simulink model "MBDMotorSystemModel"  (R2023a)
settings: Solver=VariableStepAuto  StartTime=0.0  StopTime=1  RelTol=1e-3
undefined symbols (not defined in the file): CntFdqDcpMap, CntLdqDMap, CntTrqReqMap, DiscIntNeverNeededParam, MdlFluxMap, MdlTrqMap, Pos0
libraries: simulink x29, simulink_extras x6
(part 1 of 3)
settings Model: SimulationMode=accelerator  Creator=DevMDG39khtN  LastModifiedBy=DevMDG39khtN

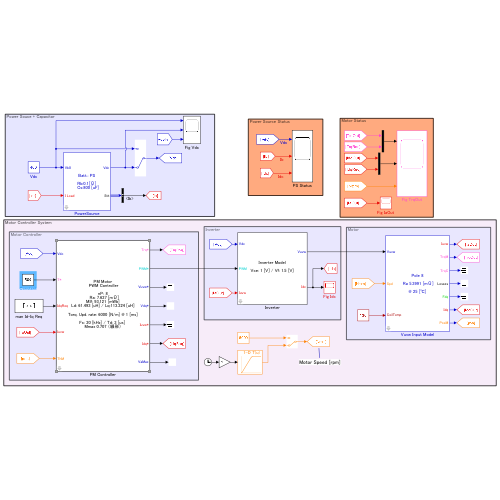
[thumbnail: Simulink's stored preview of the top-level diagram]
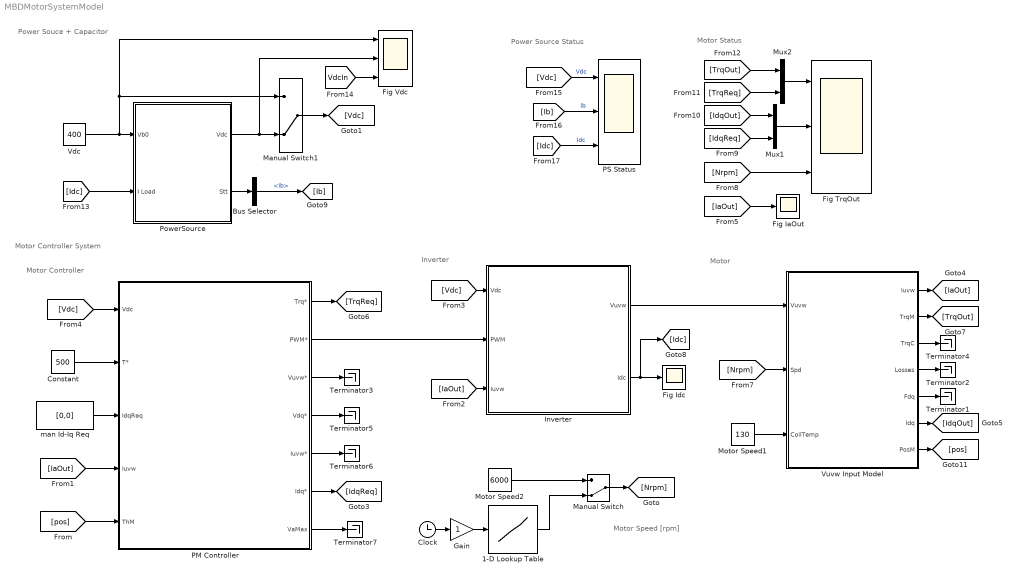
== system MBDMotorSystemModel ==
  note: Motor Speed [rpm]
  note: Power Source Status
  note: Motor Controller System
  note: Motor Controller
  note: Inverter
  note: Motor
  note: Motor Status
  note: Power Souce + Capacitor
  1-D Lookup Table : Lookup_n-D  NumberOfTableDimensions=1  BreakpointsForDimension1=[0 0.01 0.4 0.45 0.8]  Table=[0 0 12000 13000 13000]  InternalRulePriority=Speed  RndMeth=Simplest
  Bus Selector : BusSelector  OutputSignals=Ib
  Clock : Clock
  Constant : Constant  Value=500
  Fig IaOut : Scope
  Fig Idc : Scope
  Fig TrqOut : Scope  NumInputPorts=3
  Fig Vdc : Scope  NumInputPorts=3
  Gain : Gain
  Inverter : Subsystem  mask{Vce=1, Vf=1.5}
      mask prompts: Vce "Vce Sw On Vlotage[V]"; Vf "Vf FWD On Vlotage[V]"
      mask TypeOptions Vce: Voltage 3Phase/Vce
      mask TypeOptions Vf: Voltage 3Phase/Vf
      mask Display:
      | disp( [ ...
      |     'Inverter Model\n\n', ...
      |     sprintf('Vce: %g [V] / Vf: %g [V]\n',Vce,Vf), ...
      |     ]);
  Manual Switch : ManualSwitch  CurrentSetting=0
  Manual Switch1 : ManualSwitch  CurrentSetting=0
  Motor Speed1 : Constant  Value=130
  Motor Speed2 : Constant  Value=6000
  Mux1 : Mux  Inputs=2
  Mux2 : Mux  Inputs=2
  PM Controller : Subsystem  mask{MapTrqToIdq=CntTrqReqMap, MapLimitTrq=CntTrqReqMap.Limit.TrqMaxIa, DltTrqLmt=6000, TsTrqUpdM=1, KcDt=3000, KcQt=3000, KcDw=1500, KcQw=1500, IsLinPGain=off, IsLdqRef=on, IsDcpRef=on, MapVdcpl=CntFdqDcpMap, MapDynLdq=CntLdqDMap, nP=8, RaM=7.627, MIfM=93.121, LdU=61.493, LqU=113.224, IaRange=1200, IanBit=12, IaIsClamp=on, TssU=100, tauMs=2, Nmw=8, RnBit=12, nX=4, TsvU=100, tauMv=4, MaxVdc=600, MinVdc=0, VnBit=10, VIsClamp=on, FcK=20, TdU=3, IsDeadTimeCorrection=on, IsTdIaReq=on, vThr=0, TypePWMVz=0:SVM, lMaxVdc=0.707 （線形）, IsOvrMod=on}
      mask prompts: MapTrqToIdq "トルク⇒電流指令マップ"; MapLimitTrq "トルク制限マップ"; DltTrqLmt "トルク変化率 [Nm/s]"; TsTrqUpdM "トルク更新周期 [ms]"; KcDt "d軸 Cut off Gain [rad./s]"; KcQt "q軸 Cut off Gain [rad./s]"; KcDw "d軸 Cut off Gain [rad./s]"; KcQw "q軸 Cut off Gain [rad./s]"; IsLinPGain "比例ゲイン固定"; IsLdqRef "Ldq マップ 電流指令値参照"; IsDcpRef "非干渉化マップ 電流指令値参照"; MapVdcpl "非干渉化マップ"; MapDynLdq "インダクタンスマップ"; nP "極数"; RaM "電機子抵抗 [mΩ]"; MIfM "磁石鎖交磁束 [mWb]"; LdU "d軸インダクタンス [uH]"; LqU "q軸インダクタンス [uH]"; IaRange "Current Range [A]"; IanBit "Quantization Bit"; IaIsClamp "Out of Range Clamp"; TssU "Sample Period [us]"; tauMs "LPF Time Constant [ms]"; Nmw "Moving Average Num"; RnBit "R/D Quant. Bit"; nX "Resolver X num."; TsvU "Sample period [us]"; tauMv "LPF Time Constant [ms]"; MaxVdc "Max. Volt. Range [V]"; MinVdc "Min. Volt. Range [V]"; VnBit "Quantization Bit"; VIsClamp "Out of Range Clamp"; FcK "Carrier Freq.  [kHz]"; TdU "DeadTime [us]"; IsDeadTimeCorrection "DeadTime Correction"; IsTdIaReq "Use Command"; vThr "補償方向電流閾値"; TypePWMVz "PWM Vz"; lMaxVdc "最大電圧利用率"; IsOvrMod "過変調補正有効"
      mask init:
      | TsTrqUpd = TsTrqUpdM*1e-3;
      |     
      |     if strcmp(get_param(gcbh,'IsTdIaReq'),'on')
      |         fIaReq=1;
      |     else
      |         fIaReq=0;
      |     end    
      | 
      |     vdMapD   = MapVdcpl.Map.D;
      |     vdMapQ   = MapVdcpl.Map.Q;
      |     axIdX    = MapVdcpl.Axis.Id;
      |     axIqY    = MapVdcpl.Axis.Iq;
      | 
      |     ldMapD   = MapDynLdq.Map.D;
      |     ldMapQ   = MapDynLdq.Map.Q;
      |     axIdXL   = MapDynLdq.Axis.Id;
      |     axIqYL   = MapDynLdq.Axis.Iq;
      | 
      |     VdcIdx   = MapTrqToIdq.Axis.zVdc;
      |     TrqIdx   = MapTrqToIdq.Axis.rTrq;
      |     NsIdx    = MapTrqToIdq.Axis.cNrpm;
      |     IdMap    = MapTrqToIdq.Map.D;
      |     IqMap    = MapTrqToIdq.Map.Q;
      |    
      |     set_param( ...
      |         getSimulinkBlockHandle([gcb,'/Fc']), 'Value', ...
      |         num2str(evalin('base', get_param(gcbh,'FcK'))))
      mask TypeOptions DltTrqLmt:
      | IPM
      | Trq To Id-Iq Request/DltTrqLmt
      mask TypeOptions IsLinPGain:
      | PM Feedback
      |  Controller/IsLinPGain
      mask TypeOptions IsLdqRef:
      | PM Feedback
      |  Controller/IsLdqRef
      mask TypeOptions IsDcpRef:
      | PM Feedback
      |  Controller/IsDcpRef
      mask TypeOptions nP:
      | Resolver
      | To Elec. Pos/nP | IPM
      | Trq To Id-Iq Request/nP
      mask TypeOptions RaM:
      | PM Feedback
      |  Controller/RaM
      mask TypeOptions MIfM:
      | PM Feedback
      |  Controller/MIfM
      mask TypeOptions LdU:
      | PM Feedback
      |  Controller/LdU
      mask TypeOptions LqU:
      | PM Feedback
      |  Controller/LqU
      mask TypeOptions IaRange:
      | Current
      | Settings/IaRange
      mask TypeOptions IanBit:
      | Current
      | Settings/nBit
      mask TypeOptions IaIsClamp:
      | Current
      | Settings/IsClamp
      mask TypeOptions TssU: CalcFreq/TsU
      mask TypeOptions tauMs: CalcFreq/tauM
      mask TypeOptions Nmw: CalcFreq/Nmw
      mask TypeOptions RnBit: Resolver Settings/nBit
      mask TypeOptions nX: Resolver Settings/nX
      mask TypeOptions TsvU: LPF/TsU
      mask TypeOptions tauMv: LPF/tauM
      mask TypeOptions MaxVdc:
      | Voltage Settings
      |  /MaxVdc
      mask TypeOptions MinVdc:
      | Voltage Settings
      |  /MinVdc
      mask TypeOptions VnBit:
      | Voltage Settings
      |  /nBit
      mask TypeOptions VIsClamp:
      | Voltage Settings
      |  /IsClamp
      mask TypeOptions TdU: PWM Timer/TdU
      mask TypeOptions IsDeadTimeCorrection: PWM Timer/IsDeadTimeCorrection
      mask TypeOptions vThr: PWM Timer/vThr
      mask TypeOptions TypePWMVz: Modulator/TypePWMVz
      mask TypeOptions lMaxVdc:
      | PM Feedback
      |  Controller/lMaxVdc
      mask TypeOptions IsOvrMod: Modulator/IsOvrMod
      mask DialogControl Container20 Prompt: トルク⇒電流指令変換
      mask DialogControl Container17 Prompt: トルク変化率設定
      mask DialogControl Container14 Prompt: 制御パラメータ
      mask DialogControl Container18 Prompt: 電流フィードバック設定
      mask DialogControl Container19 Prompt: MTPA領域
      mask DialogControl Container19_copy Prompt: 電圧飽和領域
      mask DialogControl Container12 Prompt: モータパラメータ
      mask DialogControl Container16 Prompt: Sensor Definition
      mask DialogControl Container21 Prompt: Current Sensor
      mask DialogControl Container15 Prompt: Position Sensor
      mask DialogControl Container22 Prompt: Resolver
      mask DialogControl Container13 Prompt: Voltage Sensor
      mask DialogControl Container10 Prompt: PWM Definition
      mask DialogControl Container11 Prompt: DeadTime Def.
      mask Display:
      | disp( [ ...
      |     'PM Motor\n PWM Controller\n', ...
      |     sprintf('\nnP: %d\n  Ra: %g [mΩ]\n',nP,RaM), ...
      |     sprintf('MIf: %g [mWb]\n',MIfM) ...
      |     sprintf('Ld: %g [uH] / Lq:%g [uH]\n',LdU,LqU) ...
      |     sprintf('\nTorq. Upd. rate: %g [N/m] @ %g [ms]\n',DltTrqLmt,TsTrqUpdM) ...
      |     sprintf('\nFc: %g [kHz] / Td: %g [us] \n',FcK,TdU) ...
      |     sprintf('Mmax %s\n',get_param(gcbh,'lMaxVdc')), ...
      |     ]);
      |     % sprintf('\nKcD: %g / KcQ: %g [rad./s]\n',KcD,KcQ), ...
  PS Status : Scope  NumInputPorts=3
  PowerSource : Subsystem  mask{TypePS=PS, Rb=0.1, Cb=30, CsU=800}
      mask prompts: TypePS "PowerSource"; Rb "内部抵抗 [Ω]"; Cb "容量 [F]"; CsU "容量 [uF]"
      mask init:
      | ses = get_param(gcb,'MaskEnables');
      |     if strcmpi(get_param(gcbh, "TypePS"), 'PS')
      |         ses{3} = 'off';
      |     else
      |         ses{3} = 'on';
      |     end
      |     set_param(gcbh, 'MaskEnables', ses);
      mask TypeOptions TypePS: Source/LabelModeActiveChoice
      mask Callback TypePS:
      | ses = get_param(gcb,'MaskEnables');
      | if strcmpi(get_param(gcbh, "TypePS"), 'PS')
      |     ses{3} = 'off';
      | else
      |     ses{3} = 'on';
      | end
      | set_param(gcbh, 'MaskEnables', ses);
      mask TypeOptions Rb: Rb/Value
      mask TypeOptions Cb: Cb/Value
      mask TypeOptions CsU: Cs/Value
      mask DialogControl ParameterGroupVar Prompt: パラメーター
      mask DialogControl Container4 Prompt: Battery
      mask DialogControl EcpInfo Prompt: Capacitor
      mask DialogControl Container5 Prompt: Capacitor
      mask Display:
      | ss = get_param(gcbh, "TypePS");
      | if ~strcmpi(ss, 'PS')
      |     ss = sprintf('%s %s [F]', ss, get_param(gcbh, "Cb"));
      | end
      | ss = sprintf('%s\n\nRb:%s[Ω]', ss, get_param(gcbh,'Rb'));
      | ss = sprintf('%s\n  Cs:%s [uF]', ss, get_param(gcbh,'CsU'));
      | fprintf('Batt.: %s', ss)
      | 
      | ses = get_param(gcb,'MaskEnables');
      | if strcmpi(get_param(gcbh, "TypePS"), 'PS')
      |     ses{3} = 'off';
      | else
      |     ses{3} = 'on';
      | end
      | set_param(gcbh, 'MaskEnables', ses);
  Terminator{1..7} (7 alike) : Terminator
  Vdc : Constant  Value=400
  Vuvw Input Model : Subsystem  mask{nPole=8, Ra0=5.3991e-3, MapIdqFromFdq=MdlFluxMap, MapTrqFromIdq=MdlTrqMap, KtC=0.00393, TC0=25}
      mask prompts: nPole "Number of Pole"; Ra0 "Coil Registance [Ohm]"; MapIdqFromFdq "Flux dq -> Idq Map"; MapTrqFromIdq "Idq -> Torque Map"; KtC "Coefficient"; TC0 "Base Temp. [deg.]"
      mask TypeOptions nPole: SpdToPos/nPole | Output Torque /nPole
      mask TypeOptions Ra0: Base Ra/Value
      mask DialogControl Container3 Prompt: Motor Parameter
      mask DialogControl Container11 Prompt: Non Linear Maps
      mask DialogControl Container5 Prompt: Temp. Correction
      mask DialogControl Container6 Prompt: Coil
      mask Display: fprintf('Pole %d\n\n Ra %g [mΩ]\n\n @ %s [℃] ',nPole, Ra0*1000,get_param(gcbh,'TC0') )
  man Id-Iq Req : Constant  Value=[0,0]
  wires:
  [pos] -> PM Controller/5(ThM)
  Vuvw Input Model/1(Iuvw) -> [IaOut]
  [IaOut] -> PM Controller/4(Iuvw)
  Vuvw Input Model/4(Losses) -> Terminator2/1
  Vuvw Input Model/5(Fdq) -> Terminator1/1
  Vuvw Input Model/6(Idq) -> [IdqOut]
  Vuvw Input Model/3(TrqC) -> Terminator4/1
  Motor Speed1/1 -> Vuvw Input Model/3(CoilTemp)
  [IaOut] -> Inverter/3(Iuvw)
  [Vdc] -> Inverter/1(Vdc)
  [Vdc] -> PM Controller/1(Vdc)
  man Id-Iq Req/1 -> PM Controller/3(IdqReq)
  PM Controller/2(PWM*) -> Inverter/2(PWM)
  Inverter/2(Idc) -> Fig Idc/1, [Idc]
  Constant/1 -> PM Controller/2(T*)
  [Nrpm] -> Vuvw Input Model/2(Spd)
  Motor Speed2/1 -> Manual Switch/1
  1-D Lookup Table/1 -> Manual Switch/2
  Inverter/1(Vuvw) -> Vuvw Input Model/1(Vuvw)
  Manual Switch/1 -> [Nrpm]
  [Nrpm] -> Fig TrqOut/3
  PM Controller/6(Idq*) -> [IdqReq]
  Mux1/1 -> Fig TrqOut/2
  [IdqOut] -> Mux1/1
  [IdqReq] -> Mux1/2
  Mux2/1 -> Fig TrqOut/1
  PM Controller/1(Trq*) -> [TrqReq]
  [TrqReq] -> Mux2/2
  [TrqOut] -> Mux2/1
  Vuvw Input Model/2(TrqM) -> [TrqOut]
  PM Controller/3(Vuvw*) -> Terminator3/1
  PM Controller/4(Vdq*) -> Terminator5/1
  PM Controller/5(Iuvw*) -> Terminator6/1
  PM Controller/7(VaMax) -> Terminator7/1
  Vuvw Input Model/7(PosM) -> [pos]
  [Vdc] -> PS Status/1  "Vdc"
  [Ib] -> PS Status/2  "Ib"
  [Idc] -> PS Status/3  "Idc"
  Vdc/1 -> PowerSource/1(Vb0), Fig Vdc/1, Manual Switch1/1
  [VdcIn] -> Fig Vdc/3
  PowerSource/1(Vdc) -> Fig Vdc/2, Manual Switch1/2
  Bus Selector/1 -> [Ib]  "<Ib>"
  [IaOut] -> Fig IaOut/1
  PowerSource/2(Stt) -> Bus Selector/1
  [Idc] -> PowerSource/2(I Load)
  Manual Switch1/1 -> [Vdc]
  Clock/1 -> Gain/1
  Gain/1 -> 1-D Lookup Table/1

== system MBDMotorSystemModel/Inverter ==
  note: 0:Normal
      | 1:Short
      | 2:Open
      |
      | ※ Ignore
      | up and down short
      | at the same time.
  note: Fail State
  Vdc : Inport
  PWM : Inport  Port=2  PortDimensions=6
  Iuvw : Inport  Port=3  PortDimensions=3
  Bus Creator : BusCreator  Inputs=2
  Bus Creator1 : BusCreator  Inputs=2
  Bus Creator2 : BusCreator  Inputs=2
  Bus Creator3 : BusCreator  Inputs=3
  Constant{1..6} (6 alike) : Constant  Value=0
  DC Current : Subsystem
  Fail Process : Subsystem  mask{Vce=Vce, Vf=Vf}
      mask prompts: Vce "Vce Sw On Vlotage[V]"; Vf "Vf  FWD On Vlotage[V]"
      mask TypeOptions Vce: Vce/Value
      mask TypeOptions Vf: Vf/Value
      mask DialogControl ParameterGroupVar Prompt: パラメーター
  IdcOut : Scope
  Va PWM : Scope  NumInputPorts=3
  Voltage 3Phase : Subsystem  mask{Vce=Vce, Vf=Vf}
      mask prompts: Vce "Vce Sw On Vlotage[V]"; Vf "Vf  FWD On Vlotage[V]"
      mask TypeOptions Vce: Vce/Value
      mask TypeOptions Vf: Vf/Value
  Vuvw : Outport
  Idc : Outport  Port=2
  wires:
  Vdc/1 -> Voltage 3Phase/1(Vdc), Fail Process/2(Vdc)
  DC Current/1(Idc) -> IdcOut/1, Idc/1
  Voltage 3Phase/1(Vuvw) -> Fail Process/1(Vuvw*)
  PWM/1 -> DC Current/1(sPWM), Va PWM/2, Voltage 3Phase/2(sPWM)
  Iuvw/1 -> DC Current/2(Iuvw), Va PWM/3, Voltage 3Phase/3(Iuvw), Fail Process/3(Iuvw)
  Fail Process/1(Vuvw) -> Va PWM/1, Vuvw/1
  Bus Creator1/1 -> Bus Creator3/2  "Sv"
  Bus Creator2/1 -> Bus Creator3/3  "Sw"
  Bus Creator/1 -> Bus Creator3/1  "Su"
  Constant5/1 -> Bus Creator2/1  "up"
  Constant3/1 -> Bus Creator1/1  "up"
  Constant6/1 -> Bus Creator2/2  "dwn"
  Constant2/1 -> Bus Creator/2  "dwn"
  Constant1/1 -> Bus Creator/1  "up"
  Constant4/1 -> Bus Creator1/2  "dwn"
  Bus Creator3/1 -> [Fail]
  [Fail] -> Fail Process/4(fail Mode)

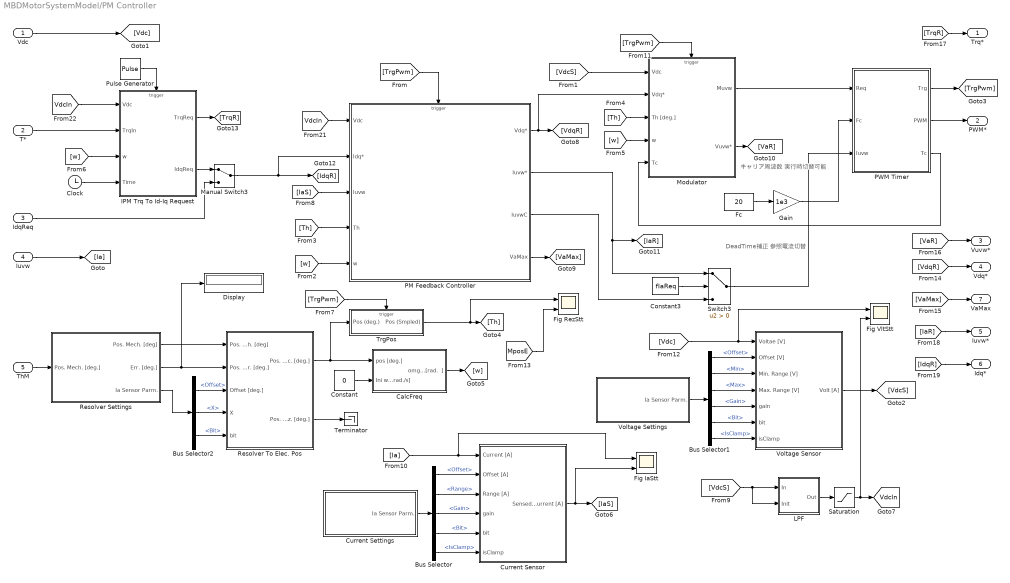
== system MBDMotorSystemModel/PM Controller ==
  note: キャリア周波数
      | 実行時切替可能
  note: DeadTime補正
      | 参照電流切替
  Vdc : Inport  PortDimensions=1
  T* : Inport  Port=2  PortDimensions=1
  IdqReq : Inport  Port=3  PortDimensions=2
  Iuvw : Inport  Port=4  PortDimensions=3
  ThM : Inport  Port=5  PortDimensions=1
  Bus Selector : BusSelector  OutputSignals=Offset,Range,Gain,Bit,IsClamp
  Bus Selector1 : BusSelector  OutputSignals=Offset,Min,Max,Gain,Bit,IsClamp
  Bus Selector2 : BusSelector  OutputSignals=Offset,X,Bit
  CalcFreq : Subsystem  mask{TsU=TssU, tauM=tauMs, Nmw=Nmw}
      mask prompts: TsU "位置検出周期 [us]"; tauM "LPF時定数 [ms]"; Nmw "速度算出移動平均サンプル数"
      mask init:
      | if Nmw  < 1 || mod(Nmw, 1) > 0
      |         error("Move Mean Num should be positive integer.")
      |     end
      |     Ts = TsU * 1e-6;
      |     tau = tauM * 1.e-3;
      |     Tw = Nmw * Ts;
      |     if Nmw > 1
      |         % set_param(gcbh,'IncludeCurrent', 'on')
      |         Ndw = Nmw-1;
      |     else
      |         % set_param(gcbh,'IncludeCurrent', 'off')
      |         Ndw = Nmw;
      |     end
  Clock : Clock
  Constant : Constant  Value=0
  Constant3 : Constant  Value=fIaReq
  Current Settings : Subsystem  mask{IaRange=IaRange, nBit=IanBit, IsClamp=on}
      mask prompts: IaRange "Current Range [A]"; nBit "Quantization Bit"; IsClamp "Out of Range Clamp"
      mask TypeOptions IaRange: Range　[A]/Value
      mask TypeOptions nBit: Bit/Value
      mask Callback IsClamp:
      | s = get_param(gcbh, 'IsClamp');
      | if strcmpi(s, 'on')
      |     set_param(sprintf('%s/IsClamp',gcb), 'Value', '1');
      | else
      |     set_param(sprintf('%s/IsClamp',gcb), 'Value', '0');
      | end
      mask DialogControl ParameterGroupVar Prompt: パラメーター
      mask DialogControl Control2 Prompt: Linear Mode if set to 0
  Current Sensor : Subsystem
  Display : Display
  Fc : Constant  Value=20
  Fig IaStt : Scope  NumInputPorts=2
  Fig RezStt : Scope  NumInputPorts=2
  Fig VltStt : Scope  NumInputPorts=2
  Gain : Gain  Gain=1e3
  IPM Trq To Id-Iq Request : Subsystem  mask{DltTrqLmt=DltTrqLmt, nP=nP, VdcIdx=VdcIdx, TrqIdx=TrqIdx, NsIdx=NsIdx, IdMap=IdMap, IqMap=IqMap, MapLmtTrq=MapLimitTrq}
      mask prompts: DltTrqLmt "トルク変化率 [Nm/s]"; nP "極数（周波数⇒回転数変換用）"; VdcIdx "DC電圧軸 [V]    (3)"; TrqIdx "トルク軸 [Nm]     (1)"; NsIdx "回転数軸 [rpm] (2)"; IdMap "d軸 電流指令マップ [A]"; IqMap "q軸 電流指令マップ [A]"; MapLmtTrq "トルク制限マップ [Nm] (Spd,Vdc)"
      mask DialogControl Container3 Prompt: トルク-dq軸電流指令変換マップ
      mask DialogControl Container5 Prompt: 軸
      mask DialogControl Container7 Prompt: マップ
  LPF : Subsystem  mask{tauM=tauMv, TsU=TsvU}
      mask prompts: tauM "時定数 [ms]"; TsU "サンプル時間 [us]"
      mask init:
      | tau = tauM * 1.0e-3;
      |     Ts = TsU * 1.e-6;
      mask DialogControl ParameterGroupVar Prompt: パラメーター
  Manual Switch3 : ManualSwitch
  Modulator : Subsystem  mask{TypePWMVz=0:SVM, IsOvrMod=on}
      mask prompts: TypePWMVz "PWM Vzタイプ"; IsOvrMod "過変調有効"
      mask init:
      | if contains(get_param(gcbh,'TypePWMVz'),'SVM')
      |         set_param(getSimulinkBlockHandle([gcb,'/TypePWM']), 'Value', '0');
      |     elseif contains(get_param(gcbh,'TypePWMVz'), 'DPWM')
      |         set_param(getSimulinkBlockHandle([gcb,'/TypePWM']), 'Value', '1');
      |     else
      |         set_param(getSimulinkBlockHandle([gcb,'/TypePWM']), 'Value', '2');
      |     end
      | 
      |     if strcmp(get_param(gcbh, 'IsOvrMod'), 'on')
      |         set_param(getSimulinkBlockHandle([gcb,'/IsOvrMod']), 'Value', '0');
      |     else
      |         set_param(getSimulinkBlockHandle([gcb,'/IsOvrMod']), 'Value', '1');
      |     end
      mask TypeOptions TypePWMVz: 0:SVM | 1:DPWM | 2:SPWM
      mask Callback TypePWMVz:
      | if contains(get_param(gcbh,'TypePWMVz'),'SVM')
      |         set_param(getSimulinkBlockHandle([gcb,'/TypePWM']), 'Value', '0');
      |     elseif contains(get_param(gcbh,'TypePWMVz'), 'DPWM')
      |         set_param(getSimulinkBlockHandle([gcb,'/TypePWM']), 'Value', '1');
      |     else
      |         set_param(getSimulinkBlockHandle([gcb,'/TypePWM']), 'Value', '2');
      |     end
      mask Callback IsOvrMod:
      | if strcmp(get_param(gcbh, 'IsOvrMod'), 'on')
      |         set_param(getSimulinkBlockHandle([gcb,'/IsOvrMod']), 'Value', '0');
      |     else
      |         set_param(getSimulinkBlockHandle([gcb,'/IsOvrMod']), 'Value', '1');
      |     end
  PM Feedback Controller : Subsystem  mask{lMaxVdc=0.707 （線形）, KcDt=KcDt, KcQt=KcQt, KcDw=KcDw, KcQw=KcQw, IsLinPGain=off, mIdqToLd=ldMapD, mIdqToLq=ldMapQ, axIdXdL=axIdXL, axIqYdL=axIqYL, IsLdqRef=on, mIdqToFd=vdMapD, mIdqToFq=vdMapQ, axIdX=axIdX, axIqY=axIqY, IsDcpRef=on, RaM=RaM, LdU=LdU, LqU=LqU, MIfM=MIfM}
      mask prompts: lMaxVdc "最大電圧利用率"; KcDt "Id Cut off Gain [rad./s]"; KcQt "Iq Cut off Gain [rad./s]"; KcDw "Id Cut off Gain [rad./s]"; KcQw "Iq Cut off Gain [rad./s]"; IsLinPGain "線形比例ゲイン"; mIdqToLd "Idq to dyn. Ld [H]"; mIdqToLq "Idq to dyn. Lq [H]"; axIdXdL "Id [A]"; axIqYdL "Iq [A]"; IsLdqRef "電流指令値参照"; mIdqToFd "Idq to Fd"; mIdqToFq "Idq to Fq"; axIdX "Id [A]"; axIqY "Iq [A]"; IsDcpRef "電流指令値参照"; RaM "電機子抵抗 [mΩ]"; LdU "d軸インダクタンス [uH]"; LqU "q軸インダクタンス [uH]"; MIfM "磁石鎖交磁束 [mWb]"
      mask init:
      | Ra  = RaM*1e-3;
      |     MIf = MIfM*1e-3;
      |     Ld  = LdU*1e-6;
      |     Lq  = LqU*1e-6;
      |     
      |     if contains(get_param(gcbh,'lMaxVdc'),'線形')
      |         kVdcU=1/sqrt(2);
      |     else
      |         kVdcU=sqrt(6)/pi;
      |     end
      | 
      |     if strcmp(get_param(gcbh,'IsDcpRef'),'on')
      |         typDcp=1;
      |     else
      |         typDcp=0;
      |     end    
      | 
      |     if strcmp(get_param(gcbh,'IsLdqRef'),'on')
      |         typLdq=1;
      |     else
      |         typLdq=0;
      |     end    
      | 
      |     if strcmp(get_param(gcbh,'IsLinPGain'),'on')
      |         typPGain=1;
      |     else
      |         typPGain=0;
      |     end
      mask TypeOptions lMaxVdc: 0.707 （線形） | 0.780（過変調）
      mask TypeOptions KcDt:
      | dq-Aixs Current Feedback
      | NonLiner Controller/KcDt
      mask TypeOptions KcQt:
      | dq-Aixs Current Feedback
      | NonLiner Controller/KcQt
      mask TypeOptions KcDw:
      | dq-Aixs Current Feedback
      | NonLiner Controller/KcDw
      mask TypeOptions KcQw:
      | dq-Aixs Current Feedback
      | NonLiner Controller/KcQw
      mask Callback IsLinPGain:
      | if strcmp(get_param(gcbh,'IsLinPGain'),'on')
      |         typPGain=1;
      |     else
      |         typPGain=0;
      |     end
      mask TypeOptions mIdqToLd: dLd Map/Table
      mask TypeOptions mIdqToLq: dLq Map/Table
      mask Callback IsLdqRef:
      | if strcmp(get_param(gcbh,'IsLdqRef'),'on')
      |         typLdq=1;
      |     else
      |         typLdq=0;
      |     end
      mask TypeOptions mIdqToFd: Fd Map/Table
      mask TypeOptions mIdqToFq: Fq Map/Table
      mask Callback IsDcpRef:
      | if strcmp(get_param(gcbh,'IsDcpRef'),'on')
      |         typDcp=1;
      |     else
      |         typDcp=0;
      |     end
      mask DialogControl Container3 Prompt: 制御パラメータ
      mask DialogControl Container7 Prompt: Fb Gain
      mask DialogControl Container5 Prompt: MTPA
      mask DialogControl Container6 Prompt: Field Weakening
      mask DialogControl Container9 Prompt: Decoupling Map
      mask DialogControl Container10 Prompt: Axis
      mask DialogControl Container11 Prompt: Dynamic Ldq Map
      mask DialogControl Container12 Prompt: Axis
      mask DialogControl Container13 Prompt: モータパラメータ
      mask Display:
      | disp(['IPM Discrete\nControler\n\n', ...
      |       sprintf('MTPA KcD:%g / KcQ:%g [rad./s]\n',KcDt,KcQt), ...
      |       sprintf(' FW  KcD:%g / KcQ:%g [rad./s]\n\n',KcDw,KcQw), ...
      |       sprintf('Mmax %s\n',get_param(gcbh,'lMaxVdc'))]);
      | 
      |       % sprintf('Ra: %g [mΩ] / MIf: %g [mWb]\n',RaM,MIfM), ...
      |       % sprintf('Ld: %g [uH] / Lq:%g [uH]\n\n',LdU,LqU) ...
  PWM Timer : Subsystem  mask{TdU=TdU, IsDeadTimeCorrection=on, vThr=vThr}
      mask prompts: TdU "DeadTime [us]"; IsDeadTimeCorrection "DeadTime補償有効"; vThr "補償方向電流閾値"
      mask init:
      | Td=TdU*1e-6;
      mask TypeOptions IsDeadTimeCorrection:
      | DeadTime
      | Correction/IsDeadTimeCorrection
      mask TypeOptions vThr:
      | DeadTime
      | Correction/vThr
      mask DialogControl Container3 Prompt: DeadTime 設定
  Pulse Generator : DiscretePulseGenerator  PulseType=Time based  Period=TsTrqUpd  PulseWidth=50
  Resolver To Elec. Pos : Subsystem  mask{nP=nP}
      mask prompts: nP "極数"
      mask init:
      | if nP< 2 || mod(nP, 1) ~= 0 || mod(nP, 2) ~= 0 
      |         error('Number of Pole should be positive and even Integer.')
      |     end
      |     Pn = nP/2;
      mask DialogControl ParameterGroupVar Prompt: パラメーター
  Resolver Settings : Subsystem  mask{nX=nX, nBit=RnBit}
      mask prompts: nX "Resolver X num."; nBit "R/D Quant. Bit"
      mask TypeOptions nX: X/Value
      mask TypeOptions nBit: Bit/Value
      mask DialogControl ParameterGroupVar Prompt: パラメーター
      mask DialogControl Control2 Prompt: Linear Mode if set to 0
  Saturation : Saturate  UpperLimit=Inf  LowerLimit=1
  Switch3 : Switch  Criteria=u2 > Threshold  SaturateOnIntegerOverflow=off  InputSameDT=off
  Terminator : Terminator
  TrgPos : Subsystem
  Voltage Sensor : Subsystem
  "Voltage Settings " : Subsystem  mask{MaxVdc=MaxVdc, MinVdc=MinVdc, nBit=VnBit, IsClamp=on}
      mask prompts: MaxVdc "Max. Volt. Range [V]"; MinVdc "Min. Volt. Range [V]"; nBit "Quantization Bit"; IsClamp "Out of Range Clamp"
      mask TypeOptions MaxVdc: Max. Range/Value
      mask TypeOptions MinVdc: Min. Range/Value
      mask TypeOptions nBit: Bit/Value
      mask Callback IsClamp:
      | s = get_param(gcbh, 'IsClamp');
      | if strcmpi(s, 'on')
      |     set_param(sprintf('%s/IsClamp',gcb), 'Value', '1');
      | else
      |     set_param(sprintf('%s/IsClamp',gcb), 'Value', '0');
      | end
      mask DialogControl ParameterGroupVar Prompt: パラメーター
      mask DialogControl Control2 Prompt: Linear Mode if set to 0
  Trq* : Outport
  PWM* : Outport  Port=2
  Vuvw* : Outport  Port=3
  Vdq* : Outport  Port=4
  Iuvw* : Outport  Port=5
  Idq* : Outport  Port=6
  VaMax : Outport  Port=7
  tag scope: VdcIn=global
  wires:
  Switch3/1 -> PWM Timer/3(Iuvw)
  PM Feedback Controller/3(IuvwC) -> Switch3/3
  PM Feedback Controller/2(Iuvw*) -> [IaR], Switch3/1
  Constant3/1 -> Switch3/2
  Fc/1 -> Gain/1
  Gain/1 -> PWM Timer/2(Fc)
  PWM Timer/2(PWM) -> PWM*/1
  Modulator/1(Muvw) -> PWM Timer/1(Req)
  Modulator/2(Vuvw*) -> [VaR]
  PM Feedback Controller/1(Vdq*) -> Modulator/2(Vdq*), [VdqR]
  IPM Trq To Id-Iq Request/1(TrqReq) -> [TrqR]
  T*/1 -> IPM Trq To Id-Iq Request/2(TrqIn)
  Pulse Generator/1 -> IPM Trq To Id-Iq Request/Trigger
  [IaS] -> PM Feedback Controller/3(Iuvw)
  PM Feedback Controller/4(VaMax) -> [VaMax]
  PWM Timer/3(Tc) -> Modulator/5(Tc)
  [VdcS] -> Modulator/1(Vdc)
  [Th] -> PM Feedback Controller/4(Th)
  [w] -> PM Feedback Controller/5(w)
  [Th] -> Modulator/3(Th [deg.])
  [w] -> Modulator/4(w)
  IdqReq/1 -> Manual Switch3/2
  IPM Trq To Id-Iq Request/2(IdqReq) -> Manual Switch3/1
  Manual Switch3/1 -> PM Feedback Controller/2(Idq*), [IdqR]
  Clock/1 -> IPM Trq To Id-Iq Request/4(Time)
  [VdcIn] -> IPM Trq To Id-Iq Request/1(Vdc)
  ThM/1 -> Resolver Settings/1(Pos. Mech. [deg.])
  Resolver Settings/3(Ia Sensor Parm.) -> Bus Selector2/1
  Bus Selector2/2 -> Resolver To Elec. Pos/4(X)  "<X>"
  Bus Selector1/5 -> Voltage Sensor/6(bit)  "<Bit>"
  Resolver To Elec. Pos/1(Pos. Elec. [deg.]) -> TrgPos/1(Pos (deg.)), CalcFreq/1(pos [deg.])
  Resolver Settings/2(Err. [deg.]) -> Display/1, Resolver To Elec. Pos/2(Pos. Err. [deg.])
  Resolver Settings/1(Pos. Mech. [deg]) -> Resolver To Elec. Pos/1(Pos. Mech. [deg])
  CalcFreq/1(omg. [rad.  ]) -> [w]
  TrgPos/1(Pos (Smpled)) -> Fig RezStt/1, [Th]
  Bus Selector2/3 -> Resolver To Elec. Pos/5(bit)  "<Bit>"
  Bus Selector1/1 -> Voltage Sensor/2(Offset [V])  "<Offset>"
  Bus Selector1/4 -> Voltage Sensor/5(gain)  "<Gain>"
  [Vdc] -> Fig VltStt/1, Voltage Sensor/1(Voltae [V])
  Bus Selector1/2 -> Voltage Sensor/3(Min. Range [V])  "<Min>"
  Bus Selector1/3 -> Voltage Sensor/4(Max. Range [V])  "<Max>"
  "Voltage Settings "/1(Ia Sensor Parm.) -> Bus Selector1/1
  Bus Selector/5 -> Current Sensor/6(isClamp)  "<IsClamp>"
  Bus Selector/1 -> Current Sensor/2(Offset [A])  "<Offset>"
  Bus Selector/4 -> Current Sensor/5(bit)  "<Bit>"
  Bus Selector/3 -> Current Sensor/4(gain)  "<Gain>"
  Bus Selector2/1 -> Resolver To Elec. Pos/3(Offset [deg.])  "<Offset>"
  Current Sensor/1(Sensed Current [A]) -> Fig IaStt/2, [IaS]
  Constant/1 -> CalcFreq/2(Ini w [rad./s])
  Bus Selector1/6 -> Voltage Sensor/7(isClamp)  "<IsClamp>"
  Bus Selector/2 -> Current Sensor/3(Range [A])  "<Range>"
  Current Settings/1(Ia Sensor Parm.) -> Bus Selector/1
  [w] -> IPM Trq To Id-Iq Request/3(w)
  [TrgPwm] -> TrgPos/Trigger
  [Ia] -> Fig IaStt/1, Current Sensor/1(Current [A])
  [TrgPwm] -> Modulator/Trigger
  [TrgPwm] -> PM Feedback Controller/Trigger
  [MposE] -> Fig RezStt/2
  [VdqR] -> Vdq*/1
  [VaMax] -> VaMax/1
  [VaR] -> Vuvw*/1
  [IaR] -> Iuvw*/1
  Iuvw/1 -> [Ia]
  [IdqR] -> Idq*/1
  PWM Timer/1(Trg) -> [TrgPwm]
  [TrqR] -> Trq*/1
  Voltage Sensor/1(Volt [A]) -> [VdcS]
  Resolver To Elec. Pos/2(Pos. Rez. [deg.]) -> Terminator/1
  Vdc/1 -> [Vdc]
  [VdcS] -> LPF/2(Init), LPF/1(In)
  [VdcIn] -> PM Feedback Controller/1(Vdc)
  LPF/1(Out) -> Saturation/1
  Saturation/1 -> Fig VltStt/2, [VdcIn]

== system MBDMotorSystemModel/PowerSource ==
  note: Batt. Capacitor
  note: Battery
  note: Capacitor
  note: Inner Status
  Vb0 : Inport
  I Load : Inport  Port=2
  Bus Creator2 : BusCreator  Inputs=5
  Cb : Constant  Value=Cb
  Cs : Constant  Value=CsU
  Divide : Product  Inputs=*/
  Divide1 : Product  Inputs=*/
  Divide2 : Product  Inputs=*/
  Gain : Gain  Gain=-1
  Gain1 : Gain  Gain=1e-6
  Integrator : Integrator  InitialConditionSource=external  LimitOutput=on  LowerSaturationLimit=0
  Integrator1 : Integrator  InitialConditionSource=external
  Rb : Constant  Value=Rb
  Source : VariantSource  VariantControlMode=label  LabelModeActiveChoice=PS  ShowConditionOnBlock=on
  Sum1 : Sum  Inputs=+-
  Sum2 : Sum  Inputs=-+
  Vdc : Outport
  Stt : Outport  Port=2
  wires:
  Sum2/1 -> Divide/1
  Integrator1/1 -> Source/2
  Vb0/1 -> Source/1, Integrator/2, Integrator1/2
  Cb/1 -> Divide1/2
  Divide/1 -> Gain/1, [Ib]
  Divide1/1 -> Integrator1/1
  Gain/1 -> Divide1/1
  Rb/1 -> Divide/2
  Source/1 -> [Vb], Sum2/2  "Vb"
  Bus Creator2/1 -> Stt/1  "EbStt"
  Integrator/1 -> Vdc/1, [Vdc]
  [Ib] -> Sum1/1
  Cs/1 -> Gain1/1
  Sum1/1 -> Divide2/1, [Ics]
  I Load/1 -> Sum1/2, [Io]
  Divide2/1 -> Integrator/1
  [Vdc] -> Sum2/1
  [Vdc] -> Bus Creator2/1  "Vdc"
  [Io] -> Bus Creator2/2  "Iload"
  [Ics] -> Bus Creator2/5  "Ics"
  [Ib] -> Bus Creator2/4  "Ib"
  [Vb] -> Bus Creator2/3  "Vb"
  Gain1/1 -> Divide2/2

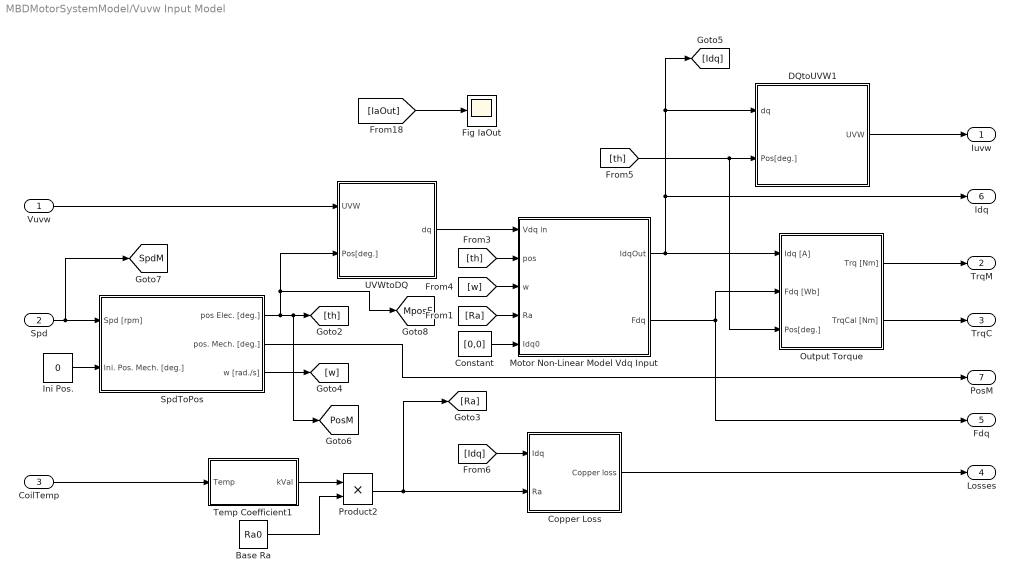
== system MBDMotorSystemModel/Vuvw Input Model ==
  Vuvw : Inport  PortDimensions=3
  Spd : Inport  Port=2
  CoilTemp : Inport  Port=3
  Base Ra : Constant  Value=Ra0
  Constant : Constant  Value=[0,0]
  Copper Loss : Subsystem
  DQtoUVW1 : Subsystem
      mask Display: fprintf('DQ to UVW');
  Fig IaOut : Scope
  Ini Pos. : Constant  Value=0
  Motor Non-Linear Model Vdq Input : Subsystem  mask{MapFdqToId=MapIdqFromFdq, MapIdq0ToFd0=MapIdqFromFdq.Ref}
      mask prompts: MapFdqToId "Flux dq -> Idq Map"; MapIdq0ToFd0 "Initial Fdq <- Idq Map"
      mask init:
      | iMapD = MapFdqToId.Map.D;
      |     iMapQ = MapFdqToId.Map.Q;
      |     yFd   = MapFdqToId.Axis.Fd;
      |     xFq   = MapFdqToId.Axis.Fq;
      |     zTh   = MapFdqToId.Axis.Theta;
      | 
      |     fMapD = MapIdq0ToFd0.Map.D;
      |     fMapQ = MapIdq0ToFd0.Map.Q;
      |     yId   = MapIdq0ToFd0.Axis.Id;
      |     xIq   = MapIdq0ToFd0.Axis.Iq;
      |     fzTh  = MapIdq0ToFd0.Axis.Theta;
      mask Display: fprintf('NonLinear\nFdq->Idq Model')
  "Output Torque " : Subsystem  mask{MapTrqFromIdq=MapTrqFromIdq, nPole=nPole}
      mask prompts: MapTrqFromIdq "Torque with Ripple [Nm]"; nPole "Number of Pole"
      mask init:
      | tMap = MapTrqFromIdq.Map;
      |     yIdT = MapTrqFromIdq.Axis.Id;
      |     xIqT = MapTrqFromIdq.Axis.Iq;
      |     zThT = MapTrqFromIdq.Axis.Theta;
      mask DialogControl Container3 Prompt: Torque Ripple Map
  Product2 : Product
  SpdToPos : Subsystem  mask{nPole=nPole}
      mask prompts: nPole "極数"
      mask init:
      | if nPole< 2 && mod(nPole, 2) ~= 0 
      |         error('Number of Pole should be positive and even.')
      |     end
      |     Pn = nPole/2;
      mask DialogControl ParameterGroupVar Prompt: パラメーター
  Temp Coefficient1 : Subsystem  mask{T0=TC0, Kt=KtC}
      mask prompts: T0 "Temp. [deg.]"; Kt "Coefficient"
      mask TypeOptions T0: BateTemp/Value
      mask TypeOptions Kt: Coefficient/Gain
      mask Display: fprintf('Temp.\nCoeff.')
  UVWtoDQ : Subsystem
      mask Display: fprintf('UVW to DQ');
  Iuvw : Outport
  TrqM : Outport  Port=2
  TrqC : Outport  Port=3
  Losses : Outport  Port=4
  Fdq : Outport  Port=5
  Idq : Outport  Port=6
  PosM : Outport  Port=7
  tag scope: MposE=global, PosM=global, SpdM=global
  wires:
  CoilTemp/1 -> Temp Coefficient1/1(Temp)
  Temp Coefficient1/1(kVal) -> Product2/1
  Base Ra/1 -> Product2/2
  [Ra] -> Motor Non-Linear Model Vdq Input/4(Ra)
  [th] -> Motor Non-Linear Model Vdq Input/2(pos)
  [w] -> Motor Non-Linear Model Vdq Input/3(w)
  UVWtoDQ/1(dq) -> Motor Non-Linear Model Vdq Input/1(Vdq in)
  Vuvw/1 -> UVWtoDQ/1(UVW)
  Motor Non-Linear Model Vdq Input/1(IdqOut) -> "Output Torque "/1(Idq [A]), Idq/1, DQtoUVW1/1(dq), [Idq]
  [th] -> DQtoUVW1/2(Pos[deg.]), "Output Torque "/3(Pos[deg.])
  DQtoUVW1/1(UVW) -> Iuvw/1
  [Idq] -> Copper Loss/1(Idq)
  Product2/1 -> Copper Loss/2(Ra), [Ra]
  Copper Loss/1(Copper loss) -> Losses/1
  Motor Non-Linear Model Vdq Input/2(Fdq) -> "Output Torque "/2(Fdq [Wb]), Fdq/1
  "Output Torque "/1(Trq [Nm]) -> TrqM/1
  "Output Torque "/2(TrqCal [Nm]) -> TrqC/1
  Constant/1 -> Motor Non-Linear Model Vdq Input/5(Idq0)
  Spd/1 -> [SpdM], SpdToPos/1(Spd [rpm])
  SpdToPos/3(w [rad./s]) -> [w]
  Ini Pos./1 -> SpdToPos/2(Ini. Pos. Mech. [deg.])
  SpdToPos/2(pos. Mech. [deg.]) -> PosM/1
  SpdToPos/1(pos Elec. [deg.]) -> [PosM], [th], [MposE], UVWtoDQ/2(Pos[deg.])
  [IaOut] -> Fig IaOut/1

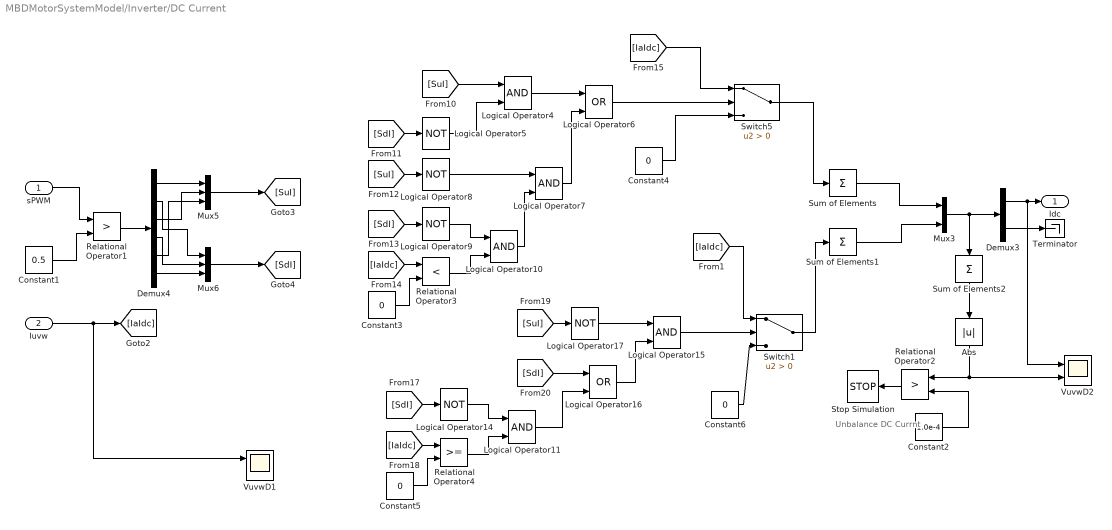
== system MBDMotorSystemModel/Inverter/DC Current ==
  note: Unbalance
      | DC Currnt
  sPWM : Inport
  Iuvw : Inport  Port=2
  Abs : Abs  ZeroCross=off  SaturateOnIntegerOverflow=off
  Constant1 : Constant  Value=0.5
  Constant2 : Constant  Value=1.0e-4
  Constant{3..6} (4 alike) : Constant  Value=0
  Demux3 : Demux  Outputs=2
  Demux4 : Demux  Outputs=6
  Logical Operator{4,7,10..11,15} (5 alike) : Logic  AllPortsSameDT=off  OutDataTypeStr=boolean
  Logical Operator{5,8..9,14,17} (5 alike) : Logic  Operator=NOT  AllPortsSameDT=off  OutDataTypeStr=boolean
  Logical Operator16 : Logic  Operator=OR  AllPortsSameDT=off  OutDataTypeStr=boolean
  Logical Operator6 : Logic  Operator=OR  AllPortsSameDT=off  OutDataTypeStr=boolean
  Mux3 : Mux  Inputs=2
  Mux5 : Mux  Inputs=3
  Mux6 : Mux  Inputs=3
  Relational Operator1 : RelationalOperator  Operator=>  OutDataTypeStr=boolean  InputSameDT=off
  Relational Operator2 : RelationalOperator  Operator=>  OutDataTypeStr=boolean  ZeroCross=off  InputSameDT=off
  Relational Operator3 : RelationalOperator  Operator=<  OutDataTypeStr=boolean  ZeroCross=off  InputSameDT=off
  Relational Operator4 : RelationalOperator  OutDataTypeStr=boolean  ZeroCross=off  InputSameDT=off
  Stop Simulation : Stop
  Sum of Elements : Sum  Inputs=+
  Sum of Elements1 : Sum  Inputs=+
  Sum of Elements2 : Sum  Inputs=+
  Switch1 : Switch  Criteria=u2 > Threshold  SaturateOnIntegerOverflow=off  InputSameDT=off
  Switch5 : Switch  Criteria=u2 > Threshold  SaturateOnIntegerOverflow=off  InputSameDT=off
  Terminator : Terminator
  VuvwD1 : Scope  NumInputPorts=2
  VuvwD2 : Scope  NumInputPorts=2
  Idc : Outport
  wires:
  Relational Operator2/1 -> Stop Simulation/1
  Abs/1 -> VuvwD2/2, Relational Operator2/1
  Constant2/1 -> Relational Operator2/2
  Logical Operator14/1 -> Logical Operator11/1
  Mux3/1 -> Demux3/1, Sum of Elements2/1
  Logical Operator5/1 -> Logical Operator4/2
  [IaIdc] -> Relational Operator4/1
  Relational Operator3/1 -> Logical Operator10/2
  Logical Operator10/1 -> Logical Operator7/2
  Relational Operator4/1 -> Logical Operator11/2
  [SdI] -> Logical Operator16/1
  [IaIdc] -> Switch5/1
  Logical Operator7/1 -> Logical Operator6/2
  Constant3/1 -> Relational Operator3/2
  [SuI] -> Logical Operator8/1
  Logical Operator9/1 -> Logical Operator10/1
  Logical Operator11/1 -> Logical Operator16/2
  Logical Operator8/1 -> Logical Operator7/1
  sPWM/1 -> Relational Operator1/1
  Logical Operator4/1 -> Logical Operator6/1
  Constant6/1 -> Switch1/3
  [IaIdc] -> Switch1/1
  Constant4/1 -> Switch5/3
  [SdI] -> Logical Operator14/1
  [SdI] -> Logical Operator5/1
  [IaIdc] -> Relational Operator3/1
  [SdI] -> Logical Operator9/1
  Constant1/1 -> Relational Operator1/2
  [SuI] -> Logical Operator4/1
  [SuI] -> Logical Operator17/1
  Constant5/1 -> Relational Operator4/2
  Switch1/1 -> Sum of Elements1/1
  Logical Operator16/1 -> Logical Operator15/2
  Switch5/1 -> Sum of Elements/1
  Logical Operator17/1 -> Logical Operator15/1
  Demux4/2 -> Mux6/1
  Demux4/4 -> Mux6/2
  Demux4/3 -> Mux5/2
  Mux5/1 -> [SuI]
  Demux4/5 -> Mux5/3
  Demux4/6 -> Mux6/3
  Relational Operator1/1 -> Demux4/1
  Mux6/1 -> [SdI]
  Demux4/1 -> Mux5/1
  Iuvw/1 -> VuvwD1/1, [IaIdc]
  Sum of Elements/1 -> Mux3/1
  Sum of Elements1/1 -> Mux3/2
  Demux3/2 -> Terminator/1
  Sum of Elements2/1 -> Abs/1
  Demux3/1 -> VuvwD2/1, Idc/1
  Logical Operator6/1 -> Switch5/2
  Logical Operator15/1 -> Switch1/2

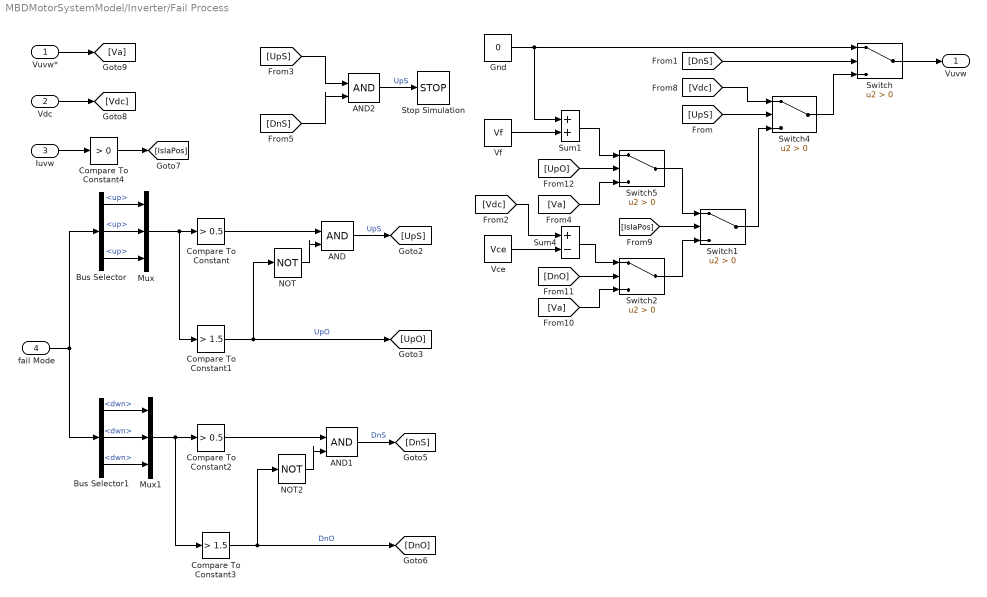
== system MBDMotorSystemModel/Inverter/Fail Process ==
  Vuvw* : Inport
  Vdc : Inport  Port=2
  Iuvw : Inport  Port=3
  fail Mode : Inport  Port=4
  AND : Logic  IconShape=distinctive  AllPortsSameDT=off  OutDataTypeStr=boolean
  AND1 : Logic  IconShape=distinctive  AllPortsSameDT=off  OutDataTypeStr=boolean
  AND2 : Logic  IconShape=distinctive  AllPortsSameDT=off  OutDataTypeStr=boolean
  Bus Selector : BusSelector  OutputSignals=Su.up,Sv.up,Sw.up
  Bus Selector1 : BusSelector  OutputSignals=Su.dwn,Sv.dwn,Sw.dwn
  Compare To Constant : simulink/Logic and Bit Operations/Compare To Constant  relop=>  const=0.5  OutDataTypeStr=boolean  ZeroCross=off
  Compare To Constant1 : simulink/Logic and Bit Operations/Compare To Constant  relop=>  const=1.5  OutDataTypeStr=boolean  ZeroCross=off
  Compare To Constant2 : simulink/Logic and Bit Operations/Compare To Constant  relop=>  const=0.5  OutDataTypeStr=boolean  ZeroCross=off
  Compare To Constant3 : simulink/Logic and Bit Operations/Compare To Constant  relop=>  const=1.5  OutDataTypeStr=boolean  ZeroCross=off
  Compare To Constant4 : simulink/Logic and Bit Operations/Compare To Constant  relop=>  const=0  OutDataTypeStr=boolean  ZeroCross=off
  Gnd : Constant  Value=0
  Mux : Mux  Inputs=3
  Mux1 : Mux  Inputs=3
  NOT : Logic  Operator=NOT  IconShape=distinctive  AllPortsSameDT=off  OutDataTypeStr=boolean
  NOT2 : Logic  Operator=NOT  IconShape=distinctive  AllPortsSameDT=off  OutDataTypeStr=boolean
  Stop Simulation : Stop
  Sum1 : Sum
  Sum4 : Sum  Inputs=+-
  Switch{,1..2,4..5} (5 alike) : Switch  Criteria=u2 > Threshold  SaturateOnIntegerOverflow=off  InputSameDT=off
  Vce : Constant  Value=Vce
  Vf : Constant  Value=Vf
  Vuvw : Outport
  wires:
  Mux/1 -> Compare To Constant1/1, Compare To Constant/1
  Compare To Constant/1 -> AND/1
  NOT/1 -> AND/2
  Compare To Constant1/1 -> [UpO], NOT/1  "UpO"
  AND/1 -> [UpS]  "UpS"
  AND1/1 -> [DnS]  "DnS"
  Compare To Constant3/1 -> [DnO], NOT2/1  "DnO"
  NOT2/1 -> AND1/2
  Compare To Constant2/1 -> AND1/1
  Mux1/1 -> Compare To Constant2/1, Compare To Constant3/1
  [DnS] -> Switch/2
  [UpS] -> Switch4/2
  Switch4/1 -> Switch/3
  Vdc/1 -> [Vdc]
  Iuvw/1 -> Compare To Constant4/1
  [IsIaPos] -> Switch1/2
  Switch2/1 -> Switch1/3
  Vuvw*/1 -> [Va]
  [DnO] -> Switch2/2
  [Va] -> Switch2/3
  Switch5/1 -> Switch1/1
  [UpO] -> Switch5/2
  Gnd/1 -> Sum1/1, Switch/1
  [Va] -> Switch5/3
  [Vdc] -> Switch4/1
  Switch1/1 -> Switch4/3
  [UpS] -> AND2/1
  [DnS] -> AND2/2
  AND2/1 -> Stop Simulation/1  "UpS"
  Switch/1 -> Vuvw/1
  fail Mode/1 -> Bus Selector1/1, Bus Selector/1
  [Vdc] -> Sum4/1
  Vce/1 -> Sum4/2
  Sum4/1 -> Switch2/1
  Sum1/1 -> Switch5/1
  Vf/1 -> Sum1/2
  Bus Selector/1 -> Mux/1  "<up>"
  Bus Selector/2 -> Mux/2  "<up>"
  Bus Selector/3 -> Mux/3  "<up>"
  Bus Selector1/1 -> Mux1/1  "<dwn>"
  Bus Selector1/2 -> Mux1/2  "<dwn>"
  Bus Selector1/3 -> Mux1/3  "<dwn>"
  Compare To Constant4/1 -> [IsIaPos]

== system MBDMotorSystemModel/Inverter/Voltage 3Phase ==
  note: Short Mode
  Vdc : Inport
  sPWM : Inport  Port=2
  Iuvw : Inport  Port=3
  Compare To Constant : simulink/Logic and Bit Operations/Compare To Constant  relop=>  const=0  OutDataTypeStr=boolean  ZeroCross=off
  Compare To Constant1 : simulink/Logic and Bit Operations/Compare To Constant  Commented=through  relop=>=  const=0.5  OutDataTypeStr=boolean
  Demux4 : Demux  Outputs=6
  Gnd : Constant  Value=0
  Logical Operator : Logic  AllPortsSameDT=off  OutDataTypeStr=boolean
  Mux5 : Mux  Inputs=3
  Mux6 : Mux  Inputs=3
  Stop Simulation : Stop
  Sum : Sum  Inputs=+-|
  Sum1 : Sum  Inputs=|++
  Sum4 : Sum  Inputs=++|
  Sum5 : Sum  Inputs=|-+
  Switch : Switch  Criteria=u2 > Threshold  SaturateOnIntegerOverflow=off  InputSameDT=off
  Switch1 : Switch  Criteria=u2 > Threshold  SaturateOnIntegerOverflow=off  InputSameDT=off
  Switch2 : Switch  Criteria=u2 > Threshold  SaturateOnIntegerOverflow=off  InputSameDT=off
  Vce : Constant  Value=Vce
  Vf : Constant  Value=Vf
  Vuvw : Outport
  wires:
  Switch1/1 -> Switch/1
  Sum/1 -> Switch1/1
  [SuP] -> Switch1/2
  Switch/1 -> Vuvw/1
  [SdP] -> Switch2/2
  Switch2/1 -> Switch/3
  Logical Operator/1 -> Stop Simulation/1
  Compare To Constant1/1 -> Demux4/1
  Demux4/1 -> Mux5/1
  Demux4/3 -> Mux5/2
  Demux4/5 -> Mux5/3
  Demux4/6 -> Mux6/3
  Demux4/4 -> Mux6/2
  Demux4/2 -> Mux6/1
  Mux5/1 -> Logical Operator/1, [SuP]
  Mux6/1 -> Logical Operator/2, [SdP]
  Iuvw/1 -> Compare To Constant/1
  Compare To Constant/1 -> Switch/2
  Vdc/1 -> Sum5/2, Sum/1
  Sum1/1 -> Switch1/3
  Vf/1 -> Sum5/1, Sum1/1
  Gnd/1 -> Sum4/1, Sum1/2
  Sum4/1 -> Switch2/1
  Sum5/1 -> Switch2/3
  Vce/1 -> Sum4/2, Sum/2
  sPWM/1 -> Compare To Constant1/1

== system MBDMotorSystemModel/PM Controller/CalcFreq ==
  pos [deg.] : Inport  SampleTime=Ts
  Ini w [rad./s] : Inport  Port=2  SampleTime=Ts
  Constant2 : Constant  Value=360
  Delay : Delay  DelayLength=1  InitialConditionSource=Input port
      settings: InputPortMap=u0,p4
  Divide1 : Product  Inputs=*/
  Divide2 : Product  Inputs=*/
  FtoW : Gain  Gain=2*pi
  Gain1 : Gain  Gain=1/360
  Gain2 : Gain  Gain=360
  Gain3 : Gain  Gain=1/180
  Gain4 : Gain  Gain=1/360
  Gain5 : Gain  Gain=1/(2*pi)
  LPF : Subsystem  mask{tauM=tauM, TsU=TsU}
      mask prompts: tauM "時定数 [ms]"; TsU "サンプル時間 [us]"
      mask init:
      | tau = tauM * 1.0e-3;
      |     Ts = TsU * 1.e-6;
      mask DialogControl ParameterGroupVar Prompt: パラメーター
  Mod1 : Math  Operator=mod
  Rounding Function : Rounding  Operator=fix
  Sample Time : Constant  Value=Ts
  Sample Time1 : Constant  Value=Tw
  Scope : Scope  Commented=on  NumInputPorts=3
  Sum : Sum  Inputs=|+-
  Sum of Elements : Sum  Inputs=+
  Sum1 : Sum  Inputs=|+-
  Tapped Delay : simulink/Discrete/Tapped Delay  vinit=0.0  samptime=-1  NumDelays=Ndw  DelayOrder=Newest  includeCurrent=on
  omg. [rad.  ] : Outport
  wires:
  Sum1/1 -> Tapped Delay/1, Divide1/1
  Sample Time/1 -> Divide1/2
  Delay/1 -> Sum/2
  Gain3/1 -> Rounding Function/1
  Gain2/1 -> Sum1/2
  Rounding Function/1 -> Gain2/1
  Divide1/1 -> Gain1/1
  pos [deg.]/1 -> Delay/1, Delay/2, Sum/1
  Tapped Delay/1 -> Sum of Elements/1
  Sum of Elements/1 -> Divide2/1
  Sample Time1/1 -> Divide2/2
  Divide2/1 -> Gain4/1
  Mod1/1 -> Gain3/1, Sum1/1
  Sum/1 -> Mod1/1
  Constant2/1 -> Mod1/2
  LPF/1(Out) -> Scope/3, FtoW/1
  Gain1/1 -> Scope/1
  Gain4/1 -> LPF/1(In), Scope/2
  Ini w [rad./s]/1 -> Gain5/1
  Gain5/1 -> [fa0]
  [fa0] -> LPF/2(Init)
  FtoW/1 -> omg. [rad.  ]/1

== system MBDMotorSystemModel/PM Controller/Current Settings ==
  note: Current Sensor Fail
  Bit : Constant  Value=nBit
  Bus Creator : BusCreator  Inputs=5
  Gain : Constant
  Gain U : Constant  Value=0
  Gain V : Constant  Value=0.2
  Gain W : Constant  Value=1.5
  IsClamp : Constant
  Manual Switch : ManualSwitch
  Manual Switch1 : ManualSwitch
  Mux : Mux  Inputs=3
  Mux1 : Mux  Inputs=3
  Offset [A] : Constant  Value=[0 0 0]
  Range　[A] : Constant  Value=IaRange
  Step : Step  Time=0.5  Before=1  After=0.3  SampleTime=0
  Step1 : Step  Time=0.8  Before=1  After=0  SampleTime=0
  Step2 : Step  Time=0.7  Before=1  After=1.5  SampleTime=0
  Ia Sensor Parm. : Outport
  wires:
  Offset [A]/1 -> Bus Creator/1  "Offset"
  Bus Creator/1 -> Ia Sensor Parm./1
  Range　[A]/1 -> Bus Creator/2  "Range"
  Bit/1 -> Bus Creator/4  "Bit"
  IsClamp/1 -> Bus Creator/5  "IsClamp"
  Gain/1 -> Manual Switch/1  "Gain"
  Step1/1 -> Mux/2
  Step/1 -> Mux/1
  Step2/1 -> Mux/3
  Manual Switch/1 -> [gain]
  [gain] -> Bus Creator/3  "Gain"
  Gain V/1 -> Mux1/2
  Gain U/1 -> Mux1/1
  Gain W/1 -> Mux1/3
  Manual Switch1/1 -> Manual Switch/2
  Mux/1 -> [gainT]
  Mux1/1 -> [GainC]
  [GainC] -> Manual Switch1/1
  [gainT] -> Manual Switch1/2

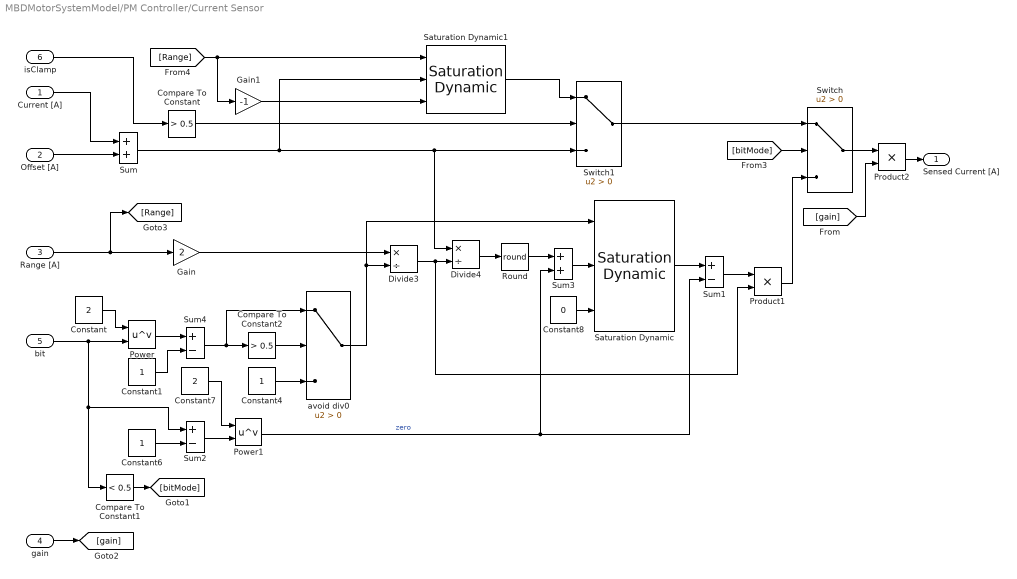
== system MBDMotorSystemModel/PM Controller/Current Sensor ==
  Current [A] : Inport  PortDimensions=3
  Offset [A] : Inport  Port=2  PortDimensions=3
  Range [A] : Inport  Port=3
  gain : Inport  Port=4
  bit : Inport  Port=5
  isClamp : Inport  Port=6
  Compare To Constant : simulink/Logic and Bit Operations/Compare To Constant  relop=>  const=0.5  OutDataTypeStr=boolean
  Compare To Constant1 : simulink/Logic and Bit Operations/Compare To Constant  relop=<  const=0.5  OutDataTypeStr=boolean
  Compare To Constant2 : simulink/Logic and Bit Operations/Compare To Constant  relop=>  const=0.5  OutDataTypeStr=boolean
  Constant : Constant  Value=2
  Constant1 : Constant
  Constant4 : Constant
  Constant6 : Constant
  Constant7 : Constant  Value=2
  Constant8 : Constant  Value=0
  Divide3 : Product  Inputs=*/
  Divide4 : Product  Inputs=*/
  Gain : Gain  Gain=2
  Gain1 : Gain  Gain=-1
  Power : Math  Operator=pow
  Power1 : Math  Operator=pow
  Product1 : Product
  Product2 : Product
  Round : Rounding  Operator=round
  Saturation Dynamic : simulink/Discontinuities/Saturation Dynamic  OutMin=[]  OutMax=[]  OutDataTypeStr=Inherit: Same as second input  OutDataType=fixdt(1, 16)  OutScaling=2^-10  DoSatur=off
  Saturation Dynamic1 : simulink/Discontinuities/Saturation Dynamic  OutMin=[]  OutMax=[]  OutDataTypeStr=Inherit: Same as second input  OutDataType=fixdt(1, 16)  OutScaling=2^-10  DoSatur=off
  Sum : Sum
  Sum1 : Sum  Inputs=+-
  Sum2 : Sum  Inputs=+-
  Sum3 : Sum
  Sum4 : Sum  Inputs=+-
  Switch : Switch  Criteria=u2 > Threshold  SaturateOnIntegerOverflow=off  InputSameDT=off
  Switch1 : Switch  Criteria=u2 > Threshold  SaturateOnIntegerOverflow=off  InputSameDT=off
  "avoid div0  " : Switch  Criteria=u2 > Threshold  SaturateOnIntegerOverflow=off  InputSameDT=off
  Sensed Current [A] : Outport
  wires:
  bit/1 -> Compare To Constant1/1, Sum2/1, Power/2
  Constant/1 -> Power/1
  Compare To Constant1/1 -> [bitMode]
  [bitMode] -> Switch/2
  Offset [A]/1 -> Sum/2
  Current [A]/1 -> Sum/1
  Power/1 -> Sum4/1
  Constant1/1 -> Sum4/2
  Sum4/1 -> Compare To Constant2/1, "avoid div0  "/1
  Range [A]/1 -> [Range], Gain/1
  Gain/1 -> Divide3/1
  Constant6/1 -> Sum2/2
  Sum2/1 -> Power1/2
  Constant7/1 -> Power1/1
  Sum/1 -> Switch1/3, Divide4/1, Saturation Dynamic1/2
  Divide3/1 -> Product1/2, Divide4/2
  Divide4/1 -> Round/1
  Power1/1 -> Sum1/2, Sum3/2  "zero"
  Sum3/1 -> Saturation Dynamic/2
  Constant8/1 -> Saturation Dynamic/3
  Saturation Dynamic/1 -> Sum1/1
  Sum1/1 -> Product1/1
  Product1/1 -> Switch/3
  isClamp/1 -> Compare To Constant/1
  Saturation Dynamic1/1 -> Switch1/1
  [Range] -> Gain1/1, Saturation Dynamic1/1
  Gain1/1 -> Saturation Dynamic1/3
  Switch1/1 -> Switch/1
  Compare To Constant/1 -> Switch1/2
  gain/1 -> [gain]
  Switch/1 -> Product2/1
  Product2/1 -> Sensed Current [A]/1
  [gain] -> Product2/2
  Round/1 -> Sum3/1
  Compare To Constant2/1 -> "avoid div0  "/2
  Constant4/1 -> "avoid div0  "/3
  "avoid div0  "/1 -> Saturation Dynamic/1, Divide3/2

== system MBDMotorSystemModel/PM Controller/IPM Trq To Id-Iq Request ==
  Vdc : Inport
  TrqIn : Inport  Port=2
  w : Inport  Port=3
  Time : Inport  Port=4
  Trigger : TriggerPort  VariantControl=Variant  PortDimensions=1
  Abs : Abs  SaturateOnIntegerOverflow=off
  Display : Display
  Gain : Gain  Gain=120/nP
  Gain1 : Gain  Gain=-1
  Id Map : Lookup_n-D  NumberOfTableDimensions=3  BreakpointsForDimension1=TrqIdx  BreakpointsForDimension2=NsIdx  BreakpointsForDimension3=VdcIdx  Table=IdMap  InternalRulePriority=Speed  RndMeth=Simplest
      settings: InputPortMap=u0,u1,u2
  Iq Map : Lookup_n-D  NumberOfTableDimensions=3  BreakpointsForDimension1=TrqIdx  BreakpointsForDimension2=NsIdx  BreakpointsForDimension3=VdcIdx  Table=IqMap  InternalRulePriority=Speed  RndMeth=Simplest
      settings: InputPortMap=u0,u1,u2
  Mux : Mux  Inputs=2
  Product : Product
  Product1 : Product
  Saturation Dynamic : simulink/Discontinuities/Saturation Dynamic  OutMin=[]  OutMax=[]  OutDataTypeStr=Inherit: Same as second input  OutDataType=fixdt(1, 16)  OutScaling=2^-10  DoSatur=off
  Scope : Scope
  Sign : Signum
  Sign1 : Signum
  Torque Rate Limitter : Subsystem  mask{DltLmt=DltTrqLmt}
      mask prompts: DltLmt "変化率制限 [unit/s]"
  Trq Limt Map : Lookup_n-D  BreakpointsForDimension1=VdcIdx  BreakpointsForDimension2=NsIdx  BreakpointsForDimension3=VdcIdx  Table=MapLimitTrq  InternalRulePriority=Speed  RndMeth=Simplest
      settings: InputPortMap=u0,u1
  WtoF : Gain  Gain=1/(2*pi)
  TrqReq : Outport
  IdqReq : Outport  Port=2
  wires:
  Mux/1 -> IdqReq/1
  Id Map/1 -> Mux/1
  w/1 -> WtoF/1
  TrqIn/1 -> Torque Rate Limitter/1(In)
  Saturation Dynamic/1 -> Product/1, Id Map/1, Iq Map/1
  Gain1/1 -> Saturation Dynamic/3
  Vdc/1 -> [Vdc]
  [Nrpm] -> Iq Map/2, Id Map/2
  Gain/1 -> Display/1, [Nrpm]
  [Vdc] -> Id Map/3, Iq Map/3
  Trq Limt Map/1 -> Scope/1, Gain1/1, Saturation Dynamic/1
  Torque Rate Limitter/1(Rate Limited) -> Abs/1, Sign1/1, Sign/1
  Time/1 -> Torque Rate Limitter/2(Time)
  Abs/1 -> Saturation Dynamic/2
  Product/1 -> TrqReq/1
  Sign/1 -> Product/2
  Product1/1 -> Mux/2
  Iq Map/1 -> Product1/1
  Sign1/1 -> Product1/2
  WtoF/1 -> Gain/1
  [Nrpm] -> Trq Limt Map/2
  [Vdc] -> Trq Limt Map/1

== system MBDMotorSystemModel/PM Controller/LPF ==
  In : Inport  SampleTime=Ts
  Init : Inport  Port=2  SampleTime=Ts
  Constant : Constant  Value=Ts
  Constant1 : Constant  Value=tau
  Delay : Delay  DelayLength=1  InitialConditionSource=Input port
      settings: InputPortMap=u0,p4
  Divide1 : Product  Inputs=*/
  Divide3 : Product  Inputs=*/
  Product : Product
  Product1 : Product
  Sum1 : Sum
  Sum2 : Sum
  Sum3 : Sum  Inputs=-+
  Out : Outport
  wires:
  Constant1/1 -> Divide1/1, Sum1/2
  Constant/1 -> Sum1/1, Divide3/1
  Sum1/1 -> Divide1/2, Divide3/2
  Divide3/1 -> [kX]
  Divide1/1 -> [kY]
  In/1 -> Product/1
  [kX] -> Product/2
  Product/1 -> Sum3/1, Sum2/1
  Sum2/1 -> Out/1, Product1/1
  [kY] -> Product1/2
  Product1/1 -> Delay/1
  Delay/1 -> Sum2/2
  Init/1 -> Sum3/2
  Sum3/1 -> Delay/2
